simulink model "III_actividad4"  (Simulink 7.9)
settings: Solver=ode45  StartTime=0.0  StopTime=2500.0  RelTol=1e-3
libraries: nintblocks x2
settings Model: Creator=root  LastModifiedBy=root
settings DebuggingCC: MaxConsecutiveZCsMsg=warning

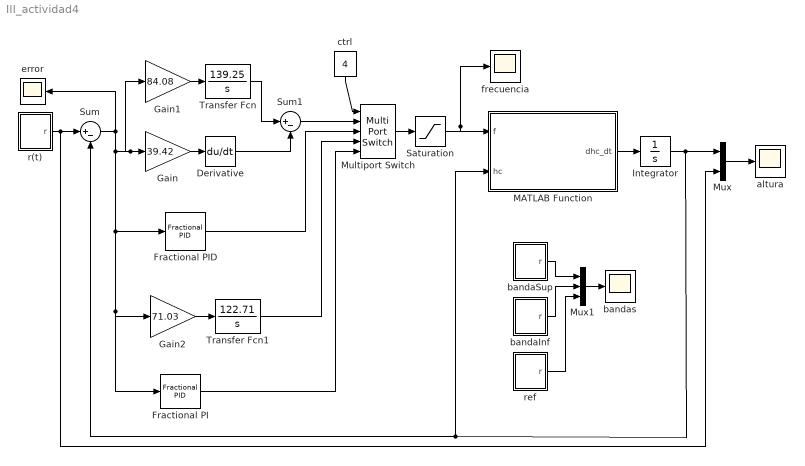
== system III_actividad4 ==
  Derivative : Derivative
  Fractional PI : nintblocks/Fractional PID  kp=71.03  kd=0  vd=1  ki=122.71  vi=-0.85  bandwidth=[0.01 100]  n=100  form1=crone  exp1=mcltime  decomp1=frac
  Fractional PID : nintblocks/Fractional PID  kp=63.29  kd=61.53  vd=0.13  ki=64.705  vi=-0.41  bandwidth=[0.01 100]  n=100  form1=crone  exp1=mcltime  decomp1=frac
  Gain : Gain  Gain=39.42
  Gain1 : Gain  Gain=84.08
  Gain2 : Gain  Gain=71.03
  Integrator : Integrator  InitialCondition=10  UpperSaturationLimit=70  LowerSaturationLimit=0
  MATLAB Function : MATLAB Function  TreatAsAtomicUnit=on
  Multiport Switch : MultiPortSwitch  Inputs=4  zeroidx=off
  Mux : Mux  Inputs=2
  Mux1 : Mux  Inputs=3
  Saturation : Saturate  UpperLimit=100  LowerLimit=0
  Sum : Sum  Inputs=|+-
  Sum1 : Sum  Inputs=|+-
  Transfer Fcn : TransferFcn  Numerator=[139.25]  Denominator=[1 0]
  Transfer Fcn1 : TransferFcn  Numerator=[122.71]  Denominator=[1 0]
  altura : Scope
      settings: TimeRange=971.6614906832298  YMin=-7.5  YMax=22.5  SaveName=hc
  bandaInf : Subsystem
  bandaSup : Subsystem
  bandas : Scope
      settings: TimeRange=971.6614906832298  YMin=14.5  YMax=22.5  SaveName=bandas
  ctrl : Constant  Value=4
  error : Scope
      settings: SaveName=error
  frecuencia : Scope
      settings: SaveName=salidaControlador
  r(t) : Subsystem
  ref : Subsystem
  wires:
  Integrator/1 -> MATLAB Function/2(hc), Sum/2, Mux/1
  Sum/1 -> error/1, Gain2/1, Fractional PI/1, Fractional PID/1, Gain/1, Gain1/1
  r(t)/1(r) -> Sum/1, Mux/2
  Saturation/1 -> frecuencia/1, MATLAB Function/1(f)
  MATLAB Function/1(dhc_dt) -> Integrator/1
  Mux/1 -> altura/1
  Gain/1 -> Derivative/1
  Multiport Switch/1 -> Saturation/1
  Sum1/1 -> Multiport Switch/2
  Derivative/1 -> Sum1/2
  Gain1/1 -> Transfer Fcn/1
  Transfer Fcn/1 -> Sum1/1
  Gain2/1 -> Transfer Fcn1/1
  Fractional PID/1 -> Multiport Switch/3
  Transfer Fcn1/1 -> Multiport Switch/4
  Fractional PI/1 -> Multiport Switch/5
  ctrl/1 -> Multiport Switch/1
  Mux1/1 -> bandas/1
  bandaSup/1(r) -> Mux1/1
  bandaInf/1(r) -> Mux1/2
  ref/1(r) -> Mux1/3

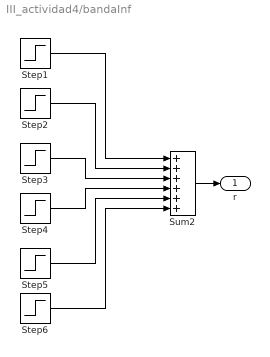
== system III_actividad4/bandaInf ==
  Step1 : Step  Time=400  Before=22.5*0.98  After=22.5*0.98  SampleTime=0
  Step2 : Step  Time=401  After=15*0.98
  Step3 : Step  Time=801  After=15*0.98
  Step4 : Step  Time=1201  After=-15*0.98
  Step5 : Step  Time=1601  After=-15*0.98
  Step6 : Step  Time=2001  After=-7.5*0.98
  Sum2 : Sum  Inputs=++++++
  r : Outport
  wires:
  Sum2/1 -> r/1
  Step1/1 -> Sum2/1
  Step2/1 -> Sum2/2
  Step5/1 -> Sum2/5
  Step6/1 -> Sum2/6
  Step3/1 -> Sum2/3
  Step4/1 -> Sum2/4

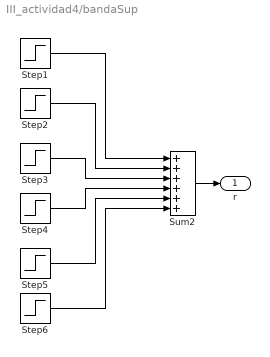
== system III_actividad4/bandaSup ==
  Step1 : Step  Time=400  Before=22.5*(1.02)  After=22.5*(1.02)  SampleTime=0
  Step2 : Step  Time=401  After=15*(1.02)
  Step3 : Step  Time=801  After=15*(1.02)
  Step4 : Step  Time=1201  After=-15*(1.02)
  Step5 : Step  Time=1601  After=-15*(1.02)
  Step6 : Step  Time=2001  After=-7.5*(1.02)
  Sum2 : Sum  Inputs=++++++
  r : Outport
  wires:
  Sum2/1 -> r/1
  Step1/1 -> Sum2/1
  Step2/1 -> Sum2/2
  Step5/1 -> Sum2/5
  Step6/1 -> Sum2/6
  Step3/1 -> Sum2/3
  Step4/1 -> Sum2/4

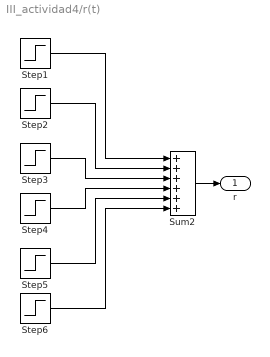
== system III_actividad4/r(t) ==
  Step1 : Step  Time=400  Before=22.5  After=22.5  SampleTime=0
  Step2 : Step  Time=401  After=15
  Step3 : Step  Time=801  After=15
  Step4 : Step  Time=1201  After=-15
  Step5 : Step  Time=1601  After=-15
  Step6 : Step  Time=2001  After=-7.5
  Sum2 : Sum  Inputs=++++++
  r : Outport
  wires:
  Sum2/1 -> r/1
  Step1/1 -> Sum2/1
  Step2/1 -> Sum2/2
  Step5/1 -> Sum2/5
  Step6/1 -> Sum2/6
  Step3/1 -> Sum2/3
  Step4/1 -> Sum2/4

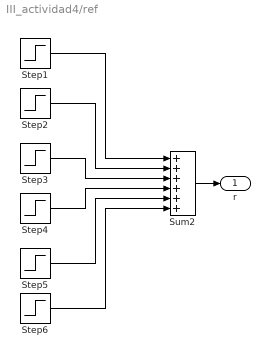
== system III_actividad4/ref ==
  Step1 : Step  Time=400  Before=22.5  After=22.5  SampleTime=0
  Step2 : Step  Time=401  After=15
  Step3 : Step  Time=801  After=15
  Step4 : Step  Time=1201  After=-15
  Step5 : Step  Time=1601  After=-15
  Step6 : Step  Time=2001  After=-7.5
  Sum2 : Sum  Inputs=++++++
  r : Outport
  wires:
  Sum2/1 -> r/1
  Step1/1 -> Sum2/1
  Step2/1 -> Sum2/2
  Step5/1 -> Sum2/5
  Step6/1 -> Sum2/6
  Step3/1 -> Sum2/3
  Step4/1 -> Sum2/4

== matlab function MATLAB Function ==
  data: f input double; dhc_dt output double; hc input double
function dhc_dt = ModeloNoLineal(f, hc)
%#codegen

    dhc_dt = (5.43*f-78.43-20.21*sqrt(abs(hc)))/(0.63*(hc.^2)+11.4*hc+17.1);
end
